simulink model "PolePlacement_Liftoff_HW_2024_lab"  (R2024b)
settings: Solver=ode1  StartTime=0.0  StopTime=inf  FixedStep=0.002  RelTol=1e-3  EnableMultiTasking=on
PostLoadFcn:
  | qc_set_target_type(getConfigSet(bdroot, 'QUARC Default Target Configuration'));
undefined symbols (not defined in the file): c_catch, HIL, Kf, P_lyap
libraries: quarc_library x4, simulink x1
settings Model: SimulationMode=external  ExtModeTrigDuration=5000  Creator=pmartin  LastModifiedBy=Student
settings SolverCC: AlgebraicLoopSolver=TrustRegion  PositivePriorityOrder=on
settings DataIOCC: LimitDataPoints=on  SaveFormat=Array  SignalLoggingSaveFormat=ModelDataLogs  ReturnWorkspaceOutputs=off
settings OptimizationCC: ExpressionDepthLimit=2147483647  InitFltsAndDblsToZero=on
settings DebuggingCC: SaveWithParameterizedLinksMsg=none  UnderspecifiedInitializationDetection=Classic  MergeDetectMultiDrivingBlocksExec=none  SolverPrmCheckMsg=warning  MultiTaskDSMMsg=warning  MultiTaskCondExecSysMsg=none  FcnCallInpInsideContextMsg=warning  UnconnectedInputMsg=warning  UnconnectedOutputMsg=warning  UnconnectedLineMsg=warning  StateNameClashWarn=warning  SFUnexpectedBacktrackingDiag=warning  SFNoUnconditionalDefaultTransitionDiag=warning  SFExecutionAtInitializationDiag=none  ArithmeticOperatorsInVariantConditions=warning
settings ModelReferenceCC: PropagateSignalLabelsOutOfModel=off
settings SFSimCC: SimUseLocalCustomCode=off  CustomCodeUndefinedFunction=UseInterfaceOnly
settings RTWCC: Description=QUARC Win64 Target Using Toolchain  SystemTargetFile=quarc_win64.tlc  TemplateMakefile=quarc_default_tmf  RTWUseLocalCustomCode=off  Toolchain=QUARC win64 | nmake (64-bit Windows)  BuildConfiguration=Faster Runs  GPUComputeCapability=3.5
settings CodeAppCC: StateflowObjectComments=on
settings STFCustomTargetCC: ConcurrentExecutionCompliant=on  GRTInterface=on  UseToolchainInfoCompliant=on  SystemTargetFile=quarc_win64.tlc
settings GRTTargetCC: TargetLangStandard=C89/C90 (ANSI)  ParMdlRefBuildCompliant=off  CompOptLevelCompliant=off  CombineOutputUpdateFcns=off  MatFileLogging=off  CPPClassGenCompliant=off  GRTInterface=on  ExtMode=on  ExtModeMexFile=quarc_comm
settings ConfigComp: CovMetricSettings=dw  CovSaveCumulativeToWorkspaceVar=on  CovSaveSingleToWorkspaceVar=on  CovExternalEMLEnable=off

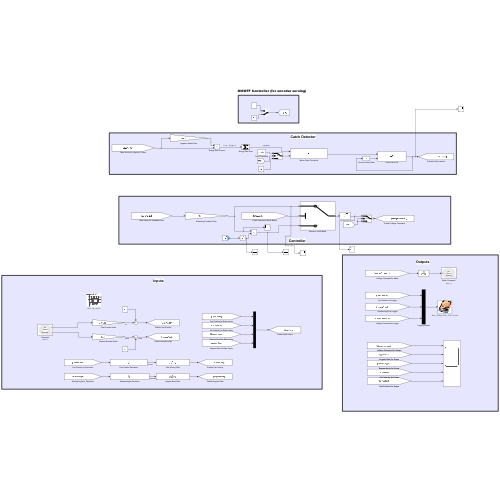
[thumbnail: Simulink's stored preview of the top-level diagram]
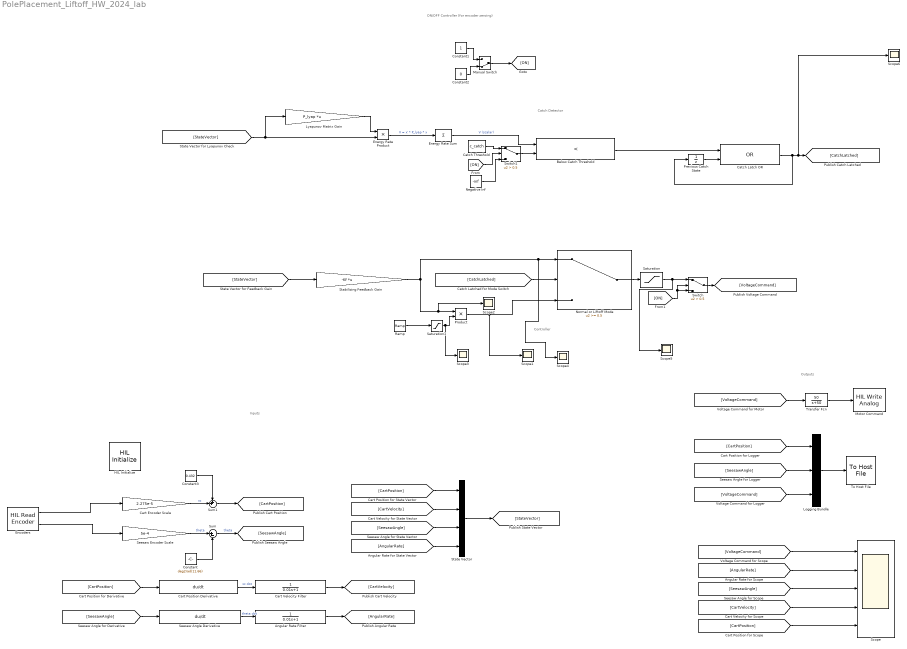
== system PolePlacement_Liftoff_HW_2024_lab ==
  note: Inputs
  note: Outputs
  note: Catch Detector
  note: ON/OFF Controller (for encoder zeroing)
  note: Controller
  Angular Rate Filter : TransferFcn  Denominator=[0.01 1]
  Below Catch Threshold : RelationalOperator  Operator=<  OutDataTypeStr=boolean  RndMeth=Simplest  InputSameDT=off
  Cart Encoder Scale : Gain  Gain=2.275e-5
  Cart Position Derivative : Derivative
  Cart Velocity Filter : TransferFcn  Denominator=[0.01 1]
  Catch Latch OR : Logic  Operator=OR  AllPortsSameDT=off  OutDataTypeStr=boolean
  Catch Threshold : Constant  Value=c_catch
  Constant : Constant  Value=deg2rad(11.66)
  Constant1 : Constant
  Constant2 : Constant  Value=0
  Constant3 : Constant  Value=0.432
  Encoders : quarc_library/Data Acquisition/Generic/Immediate I//O/HIL Read Encoder  object_name=HIL-1  channels=[0:1]  sample_time=qc_get_step_size  active=on  vector_output=off  data_type_mode=Inherit via back propagation  data_type=double
  Energy Rate Product : Product
  Energy Rate Sum : Sum  Inputs=+
  HIL Initialize : quarc_library/Data Acquisition/Generic/Configuration/HIL Initialize  object_name=HIL-1  board_type=q2_usb  board_number=0  board_options=d0=digital;d1=digital;led=auto;update_rate=normal  exclusive=off  active=off  hardware_clocks=[0:2]  clock_modes=[]  initial_clock_frequencies=[]  set_clock_params_at_start=off  set_clock_params_at_switch_in=off  set_clock_frequencies_at_start=off  set_clock_frequencies_at_switch_in=off  analog_input_channels=[0:1]  analog_input_configurations=[]  analog_input_maximums=10  analog_input_minimums=-10  set_analog_input_params_at_start=on  set_analog_input_params_at_switch_in=off  analog_output_channels=[0:1]  analog_output_maximums=10  analog_output_minimums=-10  initial_analog_outputs=[0]  final_analog_outputs=[0]  watchdog_analog_outputs=0  set_analog_output_params_at_start=on  set_analog_output_params_at_switch_in=off  set_analog_outputs_at_start=on  set_analog_outputs_at_switch_in=off  set_analog_outputs_at_terminate=on  set_analog_outputs_at_switch_out=off  set_analog_outputs_on_watchdog=off  digital_input_channels=[]  digital_output_channels=[0:7]  digital_output_configuration=[]  initial_digital_outputs=[0]  final_digital_outputs=[0]  watchdog_digital_outputs=[0]  set_digital_output_params_at_start=off  set_digital_output_params_at_switch_in=off  set_digital_outputs_at_start=on  set_digital_outputs_at_switch_in=off  set_digital_outputs_at_terminate=on  set_digital_outputs_at_switch_out=off  set_digital_outputs_on_watchdog=off  encoder_channels=[0:1]  quadrature=[4]  encoder_filter_frequency=[]  initial_encoder_counts=[0]  set_encoder_params_at_start=on  set_encoder_params_at_switch_in=off  set_encoder_counts_at_start=on  set_encoder_counts_at_switch_in=off  pwm_channels=[]  pwm_modes=[0]  pwm_frequency=1/0.020  pwm_configuration=[]  pwm_alignment=[]  pwm_polarity=[]  pwm_leading_deadband=[]  pwm_trailing_deadband=[]  initial_pwm_outputs=[0]  final_pwm_outputs=[0]  watchdog_pwm_outputs=[0]  set_pwm_params_at_start=on  set_pwm_params_at_switch_in=off  set_pwm_outputs_at_start=on  set_pwm_outputs_at_switch_in=off  set_pwm_outputs_at_terminate=on  set_pwm_outputs_at_switch_out=off  set_pwm_outputs_on_watchdog=off  other_output_channels=[]  initial_other_outputs=[]  final_other_outputs=[]  watchdog_other_outputs=[]  set_other_outputs_at_start=off  set_other_outputs_at_switch_in=off  set_other_outputs_at_terminate=off  set_other_outputs_at_switch_out=off  set_other_outputs_on_watchdog=off
  Logging Bundle : Mux  Inputs=3
  Lyapunov Matrix Gain : Gain  Gain=P_lyap  Multiplication=Matrix(K*u)
  Manual Switch : ManualSwitch  CurrentSetting=0
  Motor Command : quarc_library/Data Acquisition/Generic/Immediate I//O/HIL Write Analog  object_name=HIL-1  channels=0  sample_time=-1  active=off  vector_input=off
  Negative Inf : Constant  Value=-inf  OutDataTypeStr=Inherit: Inherit via back propagation
  Normal or Liftoff Mode : Switch  Threshold=0.5  SaturateOnIntegerOverflow=off  InputSameDT=off
  Previous Catch State : UnitDelay  SampleTime=-1
  Product : Product
  Ramp : simulink/Sources/Ramp  slope=0.3  start=0  InitialOutput=0
  Saturation : Saturate  UpperLimit=7  LowerLimit=-7
  Saturation1 : Saturate  UpperLimit=1  LowerLimit=0
  Scope : Scope  NumInputPorts=5
  Scope{1..6} (6 alike) : Scope
  Seesaw Angle Derivative : Derivative
  Seesaw Encoder Scale : Gain  Gain=5e-4
  Stabilizing Feedback Gain : Gain  Gain=-Kf  Multiplication=Matrix(K*u)
  State Vector : Mux
  Sum : Sum  Inputs=|+-
  Sum1 : Sum  Inputs=++|
  Switch : Switch  Criteria=u2 > Threshold  Threshold=0.5  SaturateOnIntegerOverflow=off  InputSameDT=off
  Switch1 : Switch  Criteria=u2 > Threshold  Threshold=0.5  SaturateOnIntegerOverflow=off  InputSameDT=off
  To Host File : quarc_library/Sinks/To Host/To Host File  source=Specify via dialog (do not evaluate)  file_name=data_%{date}_%{time}.mat  variable_name=data  decimation=1  sample_time=-1  file_format=MAT-file v.4  options=No header or footer  append=off  final_file_name=data_19-May-2026_16-01-30.mat  encoding=Default  bitrate=0
  Transfer Fcn : TransferFcn  Numerator=[50]  Denominator=[1 50]
  wires:
  [CartVelocity] -> State Vector/2
  [VoltageCommand] -> Scope/1
  [VoltageCommand] -> Transfer Fcn/1
  [CartVelocity] -> Scope/4
  [ON] -> Switch1/2
  [VoltageCommand] -> Logging Bundle/3
  [StateVector] -> Energy Rate Product/2, Lyapunov Matrix Gain/1
  Lyapunov Matrix Gain/1 -> Energy Rate Product/1
  [SeesawAngle] -> State Vector/3
  Negative Inf/1 -> Switch1/3
  Manual Switch/1 -> [ON]
  Energy Rate Sum/1 -> Below Catch Threshold/1  "V (scalar)"
  [CartPosition] -> Logging Bundle/1
  Catch Latch OR/1 -> Previous Catch State/1, Scope6/1, [CatchLatched]
  Encoders/1 -> Cart Encoder Scale/1
  Switch1/1 -> Below Catch Threshold/2
  [CartPosition] -> Cart Position Derivative/1
  State Vector/1 -> [StateVector]
  Encoders/2 -> Seesaw Encoder Scale/1
  [AngularRate] -> State Vector/4
  Angular Rate Filter/1 -> [AngularRate]
  [AngularRate] -> Scope/2
  Constant2/1 -> Manual Switch/2
  Cart Position Derivative/1 -> Cart Velocity Filter/1  "xc dot"
  Switch/1 -> [VoltageCommand]
  [ON] -> Switch/3, Switch/2
  [SeesawAngle] -> Seesaw Angle Derivative/1
  Energy Rate Product/1 -> Energy Rate Sum/1  "V = x' * P_lyap * x"
  Logging Bundle/1 -> To Host File/1
  Below Catch Threshold/1 -> Catch Latch OR/1
  Stabilizing Feedback Gain/1 -> Scope2/1, Product/1, Scope4/1, Normal or Liftoff Mode/1
  Normal or Liftoff Mode/1 -> Saturation/1
  [SeesawAngle] -> Logging Bundle/2
  Seesaw Angle Derivative/1 -> Angular Rate Filter/1  "theta dot"
  Catch Threshold/1 -> Switch1/1
  [CartPosition] -> Scope/5
  [SeesawAngle] -> Scope/3
  Cart Encoder Scale/1 -> Sum1/2  "xc"
  Constant1/1 -> Manual Switch/1
  Sum/1 -> [SeesawAngle]  "theta"
  [StateVector] -> Stabilizing Feedback Gain/1
  [CatchLatched] -> Normal or Liftoff Mode/2
  Previous Catch State/1 -> Catch Latch OR/2
  Cart Velocity Filter/1 -> [CartVelocity]
  [CartPosition] -> State Vector/1
  Transfer Fcn/1 -> Motor Command/1
  Seesaw Encoder Scale/1 -> Sum/1  "theta"
  Constant/1 -> Sum/2
  Sum1/1 -> [CartPosition]
  Constant3/1 -> Sum1/1
  Ramp/1 -> Saturation1/1
  Saturation1/1 -> Scope3/1, Product/2
  Product/1 -> Scope1/1, Normal or Liftoff Mode/3
  Saturation/1 -> Scope5/1, Switch/1
